simulink model "SVPWM"  (R2018a)
settings: Solver=VariableStepAuto  StartTime=0.0  StopTime=4  RelTol=1e-3
libraries: powerlib x12, simulink x3, electricdrivelib x1, powerlib_meascontrol x1
settings Model: Creator=Gulten  LastModifiedBy=Gulten

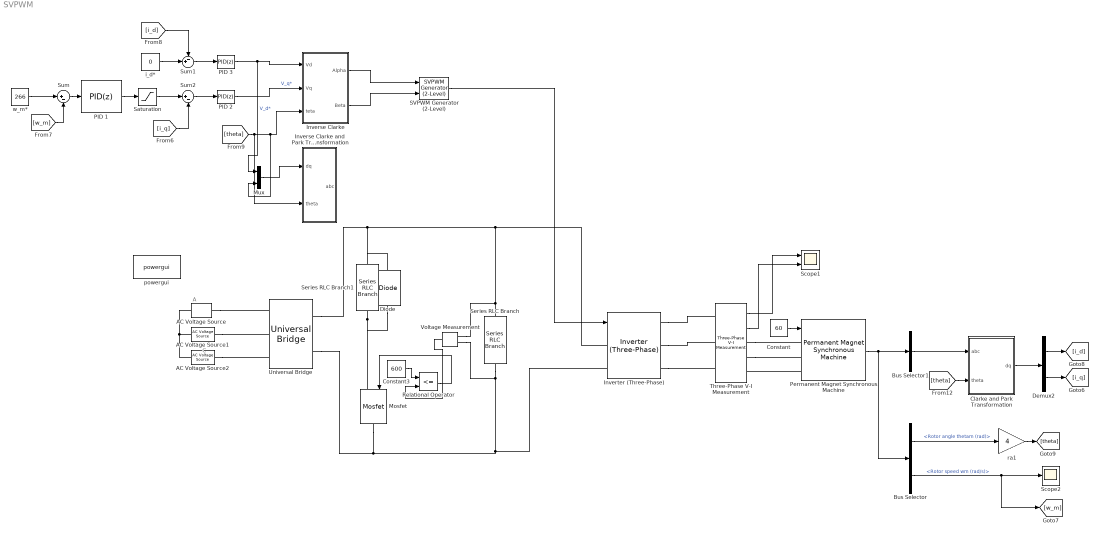
== system SVPWM ==
  note: A
  note: C
  AC Voltage Source : powerlib/Electrical Sources/AC Voltage Source  Amplitude=326.6  Phase=0  Frequency=50  SampleTime=0  Measurements=None  BusType=swing  Pref=10e3  Qref=0  Qmin=-inf  Qmax=+inf
  AC Voltage Source1 : powerlib/Electrical Sources/AC Voltage Source  Amplitude=326.6  Phase=120  Frequency=50  SampleTime=0  Measurements=None  BusType=swing  Pref=10e3  Qref=0  Qmin=-inf  Qmax=+inf
  AC Voltage Source2 : powerlib/Electrical Sources/AC Voltage Source  Amplitude=326.6  Phase=240  Frequency=50  SampleTime=0  Measurements=None  BusType=swing  Pref=10e3  Qref=0  Qmin=-inf  Qmax=+inf
  Bus Selector : BusSelector  OutputSignals=Rotor angle thetam (rad),Rotor speed wm (rad/s)
  Bus Selector1 : BusSelector  OutputSignals=Stator current is_a (A),Stator current is_b (A),Stator current is_c (A)  OutputAsBus=on
  Clarke and Park Transformation : Subsystem
  Constant : Constant  Value=60
  Constant3 : Constant  Value=600
  Demux2 : Demux  Outputs=2
  Diode : powerlib/Power Electronics/Diode  Ron=0.001  Lon=0  Vf=0.8  IC=0  UseSnubber=0  Rs=500  Cs=250e-9  Measurements=off
  Inverse Clarke : Subsystem
  Inverse Clarke and Park Transformation : Subsystem
  Inverter (Three-Phase) : electricdrivelib/Fundamental Drive Blocks/Inverter (Three-Phase)  OverrideUsingVariant=Detailed  detailLevel=Detailed  driveType=Field-oriented control  Ts=2e-6  SnubberResistance=10e3  SnubberCapacitance=inf  Device=IGBT / Diodes  Ron=1e-3  ForwardVoltages=[1.2,1.2]  GTOparameters=[1e-6,2e-6]  IGBTparameters=[1e-6,2e-6]  Measurements=All voltages and currents  converterType=Inverter  SourceFrequency=60  ReferenceFrame=Rotor  dqInductances=[8.5e-3,8.5e-3]  Inductance=8.5e-3  Ls=0  Resistance=0.2  Flux=0.175  Stator_sm=[2.01e-3,4.289e-4,4.477e-3,1.354e-3]  Stator_im=[14.85e-3,0.3027e-3]  Rotor=[9.295e-3,0.3027e-3]  Lm=10.46e-3  p=4
      settings: AttributesFormatString=%<BlockChoice>  SourceProductName=Simscape Power Systems  SourceProductBaseCode=PS
  Mosfet : powerlib/Power Electronics/Mosfet  Ron=0.1  Lon=0  Rd=0.01  Vfd=0  IC=0  Rs=1e5  Cs=inf  Measurements=off
  Mux : Mux  Inputs=2
  PID 1 : simulink/Continuous/PID Controller  Controller=PID  TimeDomain=Discrete-time  SampleTime=-1  IntegratorMethod=Forward Euler  FilterMethod=Forward Euler  Form=Parallel  UseFilter=on  ControllerParametersSource=internal  P=990  I=6  D=0  N=100  InitialConditionSource=internal  InitialConditionForIntegrator=0  InitialConditionForFilter=0  ExternalReset=none  LimitOutput=off  UpperSaturationLimit=inf  LowerSaturationLimit=-inf  LinearizeAsGain=on  AntiWindupMode=none  Kb=1  TrackingMode=off  Kt=1  PParamMin=[]  PParamMax=[]  IParamMin=[]  IParamMax=[]  DParamMin=[]  DParamMax=[]  NParamMin=[]  NParamMax=[]  KbParamMin=[]  KbParamMax=[]  KtParamMin=[]  KtParamMax=[]  POutMin=[]  POutMax=[]  IOutMin=[]  IOutMax=[]  DOutMin=[]  DOutMax=[]  NOutMin=[]  NOutMax=[]  KbOutMin=[]  KbOutMax=[]  KtOutMin=[]  KtOutMax=[]  IntegratorOutMin=[]  IntegratorOutMax=[]  FilterOutMin=[]  FilterOutMax=[]  SumOutMin=[]  SumOutMax=[]  SumI1OutMin=[]  SumI1OutMax=[]  SumI2OutMin=[]  SumI2OutMax=[]  SumI3OutMin=[]  SumI3OutMax=[]  SumDOutMin=[]  SumDOutMax=[]  SaturationOutMin=[]  SaturationOutMax=[]  IntegratorContinuousStateAttributes=''  IntegratorStateMustResolveToSignalObject=off  IntegratorRTWStateStorageClass=Auto  FilterContinuousStateAttributes=''  FilterStateMustResolveToSignalObject=off  FilterRTWStateStorageClass=Auto  DifferentiatorICPrevScaledInput=0  DifferentiatorOutMin=[]  DifferentiatorOutMax=[]  FilterDiffOutCoefMin=[]  FilterDiffOutCoefMax=[]  SumDenOutMin=[]  SumDenOutMax=[]  SumNumOutMin=[]  SumNumOutMax=[]  ReciprocalOutMin=[]  ReciprocalOutMax=[]  DivideOutMin=[]  DivideOutMax=[]  TunerSelectOption=Transfer Function Based (PID Tuner App)
  PID 2 : simulink/Continuous/PID Controller  Controller=PID  TimeDomain=Discrete-time  SampleTime=-1  IntegratorMethod=Forward Euler  FilterMethod=Forward Euler  Form=Parallel  UseFilter=on  ControllerParametersSource=internal  P=1  I=990  D=0.1  N=100  InitialConditionSource=internal  InitialConditionForIntegrator=0  InitialConditionForFilter=0  ExternalReset=none  LimitOutput=off  UpperSaturationLimit=inf  LowerSaturationLimit=-inf  LinearizeAsGain=on  AntiWindupMode=none  Kb=1  TrackingMode=off  Kt=1  PParamMin=[]  PParamMax=[]  IParamMin=[]  IParamMax=[]  DParamMin=[]  DParamMax=[]  NParamMin=[]  NParamMax=[]  KbParamMin=[]  KbParamMax=[]  KtParamMin=[]  KtParamMax=[]  POutMin=[]  POutMax=[]  IOutMin=[]  IOutMax=[]  DOutMin=[]  DOutMax=[]  NOutMin=[]  NOutMax=[]  KbOutMin=[]  KbOutMax=[]  KtOutMin=[]  KtOutMax=[]  IntegratorOutMin=[]  IntegratorOutMax=[]  FilterOutMin=[]  FilterOutMax=[]  SumOutMin=[]  SumOutMax=[]  SumI1OutMin=[]  SumI1OutMax=[]  SumI2OutMin=[]  SumI2OutMax=[]  SumI3OutMin=[]  SumI3OutMax=[]  SumDOutMin=[]  SumDOutMax=[]  SaturationOutMin=[]  SaturationOutMax=[]  IntegratorContinuousStateAttributes=''  IntegratorStateMustResolveToSignalObject=off  IntegratorRTWStateStorageClass=Auto  FilterContinuousStateAttributes=''  FilterStateMustResolveToSignalObject=off  FilterRTWStateStorageClass=Auto  DifferentiatorICPrevScaledInput=0  DifferentiatorOutMin=[]  DifferentiatorOutMax=[]  FilterDiffOutCoefMin=[]  FilterDiffOutCoefMax=[]  SumDenOutMin=[]  SumDenOutMax=[]  SumNumOutMin=[]  SumNumOutMax=[]  ReciprocalOutMin=[]  ReciprocalOutMax=[]  DivideOutMin=[]  DivideOutMax=[]  TunerSelectOption=Transfer Function Based (PID Tuner App)
  PID 3 : simulink/Continuous/PID Controller  Controller=PID  TimeDomain=Discrete-time  SampleTime=-1  IntegratorMethod=Forward Euler  FilterMethod=Forward Euler  Form=Parallel  UseFilter=on  ControllerParametersSource=internal  P=1  I=990  D=0.1  N=100  InitialConditionSource=internal  InitialConditionForIntegrator=0  InitialConditionForFilter=0  ExternalReset=none  LimitOutput=off  UpperSaturationLimit=inf  LowerSaturationLimit=-inf  LinearizeAsGain=on  AntiWindupMode=none  Kb=1  TrackingMode=off  Kt=1  PParamMin=[]  PParamMax=[]  IParamMin=[]  IParamMax=[]  DParamMin=[]  DParamMax=[]  NParamMin=[]  NParamMax=[]  KbParamMin=[]  KbParamMax=[]  KtParamMin=[]  KtParamMax=[]  POutMin=[]  POutMax=[]  IOutMin=[]  IOutMax=[]  DOutMin=[]  DOutMax=[]  NOutMin=[]  NOutMax=[]  KbOutMin=[]  KbOutMax=[]  KtOutMin=[]  KtOutMax=[]  IntegratorOutMin=[]  IntegratorOutMax=[]  FilterOutMin=[]  FilterOutMax=[]  SumOutMin=[]  SumOutMax=[]  SumI1OutMin=[]  SumI1OutMax=[]  SumI2OutMin=[]  SumI2OutMax=[]  SumI3OutMin=[]  SumI3OutMax=[]  SumDOutMin=[]  SumDOutMax=[]  SaturationOutMin=[]  SaturationOutMax=[]  IntegratorContinuousStateAttributes=''  IntegratorStateMustResolveToSignalObject=off  IntegratorRTWStateStorageClass=Auto  FilterContinuousStateAttributes=''  FilterStateMustResolveToSignalObject=off  FilterRTWStateStorageClass=Auto  DifferentiatorICPrevScaledInput=0  DifferentiatorOutMin=[]  DifferentiatorOutMax=[]  FilterDiffOutCoefMin=[]  FilterDiffOutCoefMax=[]  SumDenOutMin=[]  SumDenOutMax=[]  SumNumOutMin=[]  SumNumOutMax=[]  ReciprocalOutMin=[]  ReciprocalOutMax=[]  DivideOutMin=[]  DivideOutMax=[]  TunerSelectOption=Transfer Function Based (PID Tuner App)
  Permanent Magnet Synchronous Machine : powerlib/Machines/Permanent Magnet Synchronous Machine  NbPhases=3  FluxDistribution=Sinusoidal  RotorType=Round  MechanicalLoad=Torque Tm  PresetModel=No  ShowDetailedParameters=on  MeasurementBus=off  Resistance=50e-3  Inductance=8.5e-3  dqInductances=[500e-6,500e-6]  La=500e-6  MachineConstant=Flux linkage established by magnets (V.s)  Flux=0.2  VoltageCst=145.1039  TorqueCst=1.2  Flat=120  Mechanical=[10 0 4 0]  PolePairs=4  InitialConditions=[240,0, 0,0]  InitialConditions5ph=[266 0 0 0 0 0]  TsPowergui=0  TsBlock=-1  RefAngle=90 degrees behind phase A axis (modified Park)
      settings: SourceProductName=Simscape Power Systems
  Relational Operator : RelationalOperator  Operator=<=  OutDataTypeStr=boolean  RndMeth=Simplest
  SVPWM Generator (2-Level) : powerlib_meascontrol/Pulse & Signal Generators/SVPWM Generator (2-Level)  InputType=alpha-beta components  SwitchingPattern=Pattern #1  Fc=20000  ParUref=[0.8 -30 50]  Ts=0
      settings: SourceProductName=Simscape Power Systems  SourceProductBaseCode=PS
  Saturation : Saturate  UpperLimit=250  LowerLimit=-250
  Scope1 : Scope  NumInputPorts=2
  Scope2 : Scope
  Series RLC Branch : powerlib/Elements/Series RLC Branch  LConnTagsString=__new0  RConnTagsString=__new0  BranchType=C  Resistance=1  Inductance=1e-3  SetiL0=off  InitialCurrent=0  Capacitance=330e-3  Setx0=off  InitialVoltage=0  Measurements=None
  Series RLC Branch1 : powerlib/Elements/Series RLC Branch  LConnTagsString=__new0  RConnTagsString=__new0  BranchType=R  Resistance=5  Inductance=1e-3  SetiL0=off  InitialCurrent=0  Capacitance=1e-6  Setx0=off  InitialVoltage=0  Measurements=None
  Sum : Sum  Inputs=|+-
  Sum1 : Sum  Inputs=-+|
  Sum2 : Sum  Inputs=|+-
  Three-Phase V-I Measurement : powerlib/Measurements/Three-Phase V-I Measurement  VoltageMeasurement=phase-to-phase  SetLabelV=off  LabelV=Vabc  Vpu=off  VpuLL=off  CurrentMeasurement=yes  SetLabelI=off  LabelI=Iabc  Ipu=off  Pbase=100e6  Vbase=500e3  OutputType=Complex  PhasorSimulation=off  PSBequivalent=0
  Universal Bridge : powerlib/Power Electronics/Universal Bridge  Arms=3  SnubberResistance=1e5  SnubberCapacitance=inf  Device=Diodes  Ron=1e-3  Lon=0  ForwardVoltages="[  0  0  ]"  ForwardVoltage=0  GTOparameters=[ 10e-6 , 20e-6 ]  IGBTparameters=[ 1e-6 , 2e-6 ]  Measurements=All voltages and currents  Measurements_2=None  converterType=Rectifier
  Voltage Measurement : powerlib/Measurements/Voltage Measurement  PhasorSimulation=off  OutputType=Complex  PSBequivalent=0
  i_d* : Constant  Value=0
  powergui : powerlib/powergui  Priority=1  SimulationMode=Discrete  SampleTime=1e-6  frequency=60  Iterations=50  frequencyindice=0  Pbase=100e6  ErrMax=1e-4  UnitsV=kV  UnitsW=MW  buscounter=0  FunctionMessages=off  echomessages=off  EnableUseOfTLC=off  CurrentSourceSwitches=off  DisableSnubberDevices=off  DisableRonSwitches=off  DisableVfSwitches=off  DisplayEquations=off  SolverType=Tustin/Backward Euler (TBE)  Interpol=off  ExternalGateDelay=off  methode=off  Ts=100  x0status=blocks  SPID=on  SwTol=0  HookPort=off  RestoreLinks=warning  ResistiveCurrentMeasurement=off  Frange=[0:2:500]  Ylog=off  Xlog=on  ShowGrid=off  save=off  variable=ZData  structure=0  ZoomFFT=off  StartTime=0.0  cycles=1  DisplayStyle=1  fundamental=60  FreqAxis=off  MaxFrequency=1000  frequencyindicesteady=1  RmsSteady=1  display=off
  ra1 : Gain  Gain=4
  w_m* : Constant  Value=266
  wires:
  Constant3/1 -> Relational Operator/1
  ra1/1 -> [theta]
  Voltage Measurement/1 -> Relational Operator/2
  i_d*/1 -> Sum1/2
  PID 2/1 -> Inverse Clarke/2(Vq)  "V_q*"
  Clarke and Park Transformation/1(dq) -> Demux2/1
  Saturation/1 -> Sum2/1
  Demux2/2 -> [i_q]
  [w_m] -> Sum/2
  Sum1/1 -> PID 3/1
  [i_q] -> Sum2/2
  Demux2/1 -> [i_d]
  Sum2/1 -> PID 2/1
  Sum/1 -> PID 1/1
  PID 3/1 -> Mux/1, Inverse Clarke/1(Vd)  "V_d*"
  [theta] -> Inverse Clarke and Park Transformation/2(theta), Mux/2, Inverse Clarke/3("teta ")
  [i_d] -> Sum1/1
  Relational Operator/1 -> Mosfet/1
  Bus Selector/2 -> Scope2/1, [w_m]  "<Rotor speed wm (rad/s)>"
  Permanent Magnet Synchronous Machine/1 -> Bus Selector1/1, Bus Selector/1
  [theta] -> Clarke and Park Transformation/2(theta)
  Bus Selector1/1 -> Clarke and Park Transformation/1(abc)
  PID 1/1 -> Saturation/1
  Constant/1 -> Permanent Magnet Synchronous Machine/1
  Bus Selector/1 -> ra1/1  "<Rotor angle thetam (rad)>"
  w_m*/1 -> Sum/1
  Inverse Clarke/1(Alpha) -> SVPWM Generator (2-Level)/1
  Inverse Clarke/2(Beta) -> SVPWM Generator (2-Level)/2
  SVPWM Generator (2-Level)/1 -> Inverter (Three-Phase)/1
  Mux/1 -> Inverse Clarke and Park Transformation/1(dq)
  Three-Phase V-I Measurement/1 -> Scope1/1
  Three-Phase V-I Measurement/2 -> Scope1/2
  connections:
  Universal Bridge/RConn1 -- Diode/RConn1 -- Series RLC Branch1/LConn1 -- Inverter (Three-Phase)/LConn1 -- Series RLC Branch/LConn1 -- Voltage Measurement/LConn1
  AC Voltage Source2/LConn1 -- AC Voltage Source1/LConn1 -- AC Voltage Source/LConn1
  Universal Bridge/RConn2 -- Inverter (Three-Phase)/LConn2 -- Voltage Measurement/LConn2 -- Series RLC Branch/RConn1 -- Mosfet/RConn1
  Series RLC Branch1/RConn1 -- Diode/LConn1 -- Mosfet/LConn1
  Three-Phase V-I Measurement/RConn1 -- Permanent Magnet Synchronous Machine/LConn1
  Three-Phase V-I Measurement/RConn2 -- Permanent Magnet Synchronous Machine/LConn2
  AC Voltage Source2/RConn1 -- Universal Bridge/LConn3
  Permanent Magnet Synchronous Machine/LConn3 -- Three-Phase V-I Measurement/RConn3
  AC Voltage Source1/RConn1 -- Universal Bridge/LConn2
  AC Voltage Source/RConn1 -- Universal Bridge/LConn1
  Inverter (Three-Phase)/RConn1 -- Three-Phase V-I Measurement/LConn1
  Inverter (Three-Phase)/RConn2 -- Three-Phase V-I Measurement/LConn2
  Inverter (Three-Phase)/RConn3 -- Three-Phase V-I Measurement/LConn3

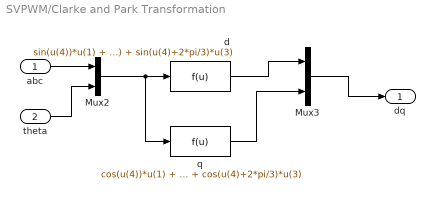
== system SVPWM/Clarke and Park Transformation ==
  abc : Inport
  theta : Inport  Port=2
  Mux2 : Mux  Inputs=2
  Mux3 : Mux  Inputs=2
  d : Fcn  Expr=sin(u(4))*u(1) + sin(u(4)-2*pi/3)*u(2) + sin(u(4)+2*pi/3)*u(3)
  q : Fcn  Expr=cos(u(4))*u(1) + cos(u(4)-2*pi/3)*u(2) + cos(u(4)+2*pi/3)*u(3)
  dq : Outport
  wires:
  q/1 -> Mux3/2
  d/1 -> Mux3/1
  theta/1 -> Mux2/2
  Mux3/1 -> dq/1
  abc/1 -> Mux2/1
  Mux2/1 -> d/1, q/1

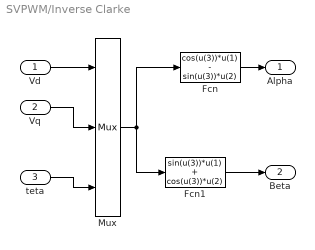
== system SVPWM/Inverse Clarke ==
  Vd : Inport
  Vq : Inport  Port=2
  "teta " : Inport  Port=3
  Fcn : Fcn  Expr=cos(u(3))*u(1) - sin(u(3))*u(2)
  Fcn1 : Fcn  Expr=sin(u(3))*u(1) + cos(u(3))*u(2)
  Mux : Mux  Inputs=3
  Alpha : Outport
  Beta : Outport  Port=2
  wires:
  Vd/1 -> Mux/1
  Fcn/1 -> Alpha/1
  Vq/1 -> Mux/2
  "teta "/1 -> Mux/3
  Mux/1 -> Fcn/1, Fcn1/1
  Fcn1/1 -> Beta/1

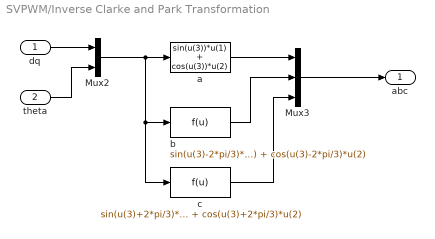
== system SVPWM/Inverse Clarke and Park Transformation ==
  dq : Inport
  theta : Inport  Port=2
  Mux2 : Mux  Inputs=2
  Mux3 : Mux  Inputs=3
  a : Fcn  Expr=sin(u(3))*u(1) + cos(u(3))*u(2)
  b : Fcn  Expr=sin(u(3)-2*pi/3)*u(1) + cos(u(3)-2*pi/3)*u(2)
  c : Fcn  Expr=sin(u(3)+2*pi/3)*u(1) + cos(u(3)+2*pi/3)*u(2)
  abc : Outport
  wires:
  theta/1 -> Mux2/2
  b/1 -> Mux3/2
  Mux2/1 -> b/1, c/1, a/1
  dq/1 -> Mux2/1
  c/1 -> Mux3/3
  Mux3/1 -> abc/1
  a/1 -> Mux3/1
